simulink model "tarot_replanning2"  (R2022a)
settings: Solver=ode45  StartTime=0.0  StopTime=sim_params.max_sim_time  FixedStep=uav.dynamics_srate  MaxStep=uav.dynamics_srate  MinStep=.005  RelTol=.005
undefined symbols (not defined in the file): constant_x_wind, constant_y_wind, constant_z_wind, DiscIntNeverNeededParam, P_failure, processes, sim_params, trajectory, uav
libraries: shared6dof x1, dspstat3 x1
(part 2 of 2)

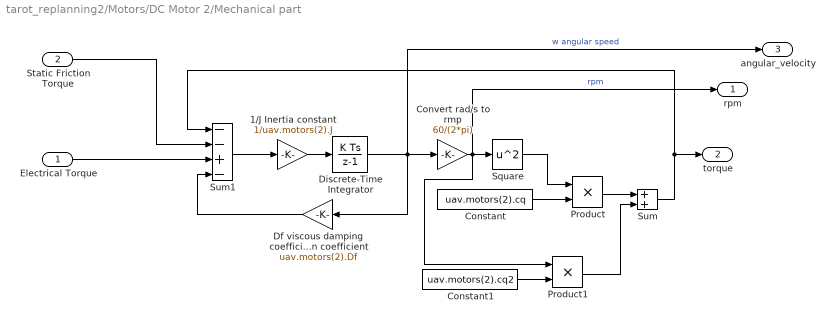
== system tarot_replanning2/Motors/DC Motor 2/Mechanical part ==
  Electrical Torque : Inport
  Static Friction Torque : Inport  Port=2
  1/J Inertia constant : Gain  Gain=1/uav.motors(2).J
  Constant : Constant  Value=uav.motors(2).cq
  Constant1 : Constant  Value=uav.motors(2).cq2
  Convert rad/s to rmp : Gain  Gain=60/(2*pi)
  "Df viscous damping coefficient Dynamic Friction coefficient " : Gain  Gain=uav.motors(2).Df
  Discrete-Time Integrator : DiscreteIntegrator  gainval=1  InitialCondition=sim_params.initial_conditions.w2  SampleTime=uav.dynamics_srate  ICPrevOutput=DiscIntNeverNeededParam  ICPrevScaledInput=DiscIntNeverNeededParam
  Product : Product
  Product1 : Product
  Square : Math  Operator=square
  Sum : Sum
  Sum1 : Sum  Inputs=--+-
  rpm : Outport  VectorParamsAs1DForOutWhenUnconnected=off
  torque : Outport  Port=2
  angular_velocity : Outport  Port=3
  wires:
  1/J Inertia constant/1 -> Discrete-Time Integrator/1
  Static Friction Torque/1 -> Sum1/2
  "Df viscous damping coefficient Dynamic Friction coefficient "/1 -> Sum1/4
  Discrete-Time Integrator/1 -> angular_velocity/1, Convert rad/s to rmp/1, "Df viscous damping coefficient Dynamic Friction coefficient "/1  "w angular speed"
  Sum1/1 -> 1/J Inertia constant/1
  Electrical Torque/1 -> Sum1/3
  Sum/1 -> Sum1/1, torque/1
  Square/1 -> Product/1
  Constant/1 -> Product/2
  Product/1 -> Sum/1
  Constant1/1 -> Product1/2
  Convert rad/s to rmp/1 -> rpm/1, Product1/1, Square/1  "rpm"
  Product1/1 -> Sum/2

== system tarot_replanning2/Motors/DC Motor 3/Electrical part ==
  ESC voltage : Inport
  w angular speed : Inport  Port=2
  1/R : Gain  Gain=1/uav.motors(3).Req
  Ke (Torque constant)1 : Gain  Gain=uav.motors(3).Ke_eq
  Kt (Torque constant) Kt=Ke for an ideal square wave motor : Gain  Gain=uav.motors(3).Ke_eq
  Saturation : Saturate  UpperLimit=uav.motors(3).current_limit  LowerLimit=0
  Sum : Sum  Inputs=|+-
  Electrical Torque : Outport  VectorParamsAs1DForOutWhenUnconnected=off
  current : Outport  Port=2  VectorParamsAs1DForOutWhenUnconnected=off
  wires:
  1/R/1 -> Saturation/1  "current i"
  Sum/1 -> 1/R/1
  Kt (Torque constant) Kt=Ke for an ideal square wave motor/1 -> Electrical Torque/1
  Ke (Torque constant)1/1 -> Sum/2
  ESC voltage/1 -> Sum/1
  w angular speed/1 -> Ke (Torque constant)1/1
  Saturation/1 -> Kt (Torque constant) Kt=Ke for an ideal square wave motor/1, current/1

== system tarot_replanning2/Motors/DC Motor 3/Mechanical part ==
  Electrical Torque : Inport
  Static Friction Torque : Inport  Port=2
  1/J Inertia constant : Gain  Gain=1/uav.motors(3).J
  Constant : Constant  Value=uav.motors(3).cq
  Constant1 : Constant  Value=uav.motors(3).cq2
  Convert rad/s to rmp : Gain  Gain=60/(2*pi)
  "Df viscous damping coefficient Dynamic Friction coefficient " : Gain  Gain=uav.motors(3).Df
  Discrete-Time Integrator : DiscreteIntegrator  gainval=1  InitialCondition=sim_params.initial_conditions.w3  SampleTime=uav.dynamics_srate  ICPrevOutput=DiscIntNeverNeededParam  ICPrevScaledInput=DiscIntNeverNeededParam
  Product : Product
  Product1 : Product
  Square : Math  Operator=square
  Sum : Sum
  Sum1 : Sum  Inputs=--+-
  rpm : Outport  VectorParamsAs1DForOutWhenUnconnected=off
  torque : Outport  Port=2
  angular_velocity : Outport  Port=3
  wires:
  1/J Inertia constant/1 -> Discrete-Time Integrator/1
  Static Friction Torque/1 -> Sum1/2
  "Df viscous damping coefficient Dynamic Friction coefficient "/1 -> Sum1/4
  Discrete-Time Integrator/1 -> angular_velocity/1, "Df viscous damping coefficient Dynamic Friction coefficient "/1, Convert rad/s to rmp/1  "w angular speed"
  Sum1/1 -> 1/J Inertia constant/1
  Electrical Torque/1 -> Sum1/3
  Sum/1 -> torque/1, Sum1/1
  Square/1 -> Product/1
  Constant/1 -> Product/2
  Product/1 -> Sum/1
  Constant1/1 -> Product1/2
  Convert rad/s to rmp/1 -> Product1/1, rpm/1, Square/1  "rpm"
  Product1/1 -> Sum/2

== system tarot_replanning2/Motors/DC Motor 4/Electrical part ==
  ESC voltage : Inport
  w angular speed : Inport  Port=2
  1/R : Gain  Gain=1/uav.motors(4).Req
  Ke (Torque constant)1 : Gain  Gain=uav.motors(4).Ke_eq
  Kt (Torque constant) Kt=Ke for an ideal square wave motor : Gain  Gain=uav.motors(4).Ke_eq
  Saturation : Saturate  UpperLimit=uav.motors(4).current_limit  LowerLimit=0
  Sum : Sum  Inputs=|+-
  Electrical Torque : Outport  VectorParamsAs1DForOutWhenUnconnected=off
  current : Outport  Port=2  VectorParamsAs1DForOutWhenUnconnected=off
  wires:
  1/R/1 -> Saturation/1  "current i"
  Sum/1 -> 1/R/1
  Kt (Torque constant) Kt=Ke for an ideal square wave motor/1 -> Electrical Torque/1
  Ke (Torque constant)1/1 -> Sum/2
  ESC voltage/1 -> Sum/1
  w angular speed/1 -> Ke (Torque constant)1/1
  Saturation/1 -> Kt (Torque constant) Kt=Ke for an ideal square wave motor/1, current/1

== system tarot_replanning2/Motors/DC Motor 4/Mechanical part ==
  Electrical Torque : Inport
  Static Friction Torque : Inport  Port=2
  1/J Inertia constant : Gain  Gain=1/uav.motors(4).J
  Constant : Constant  Value=uav.motors(4).cq
  Constant1 : Constant  Value=uav.motors(4).cq2
  Convert rad/s to rmp : Gain  Gain=60/(2*pi)
  "Df viscous damping coefficient Dynamic Friction coefficient " : Gain  Gain=uav.motors(4).Df
  Discrete-Time Integrator : DiscreteIntegrator  gainval=1  InitialCondition=sim_params.initial_conditions.w4  SampleTime=uav.dynamics_srate  ICPrevOutput=DiscIntNeverNeededParam  ICPrevScaledInput=DiscIntNeverNeededParam
  Product : Product
  Product1 : Product
  Square : Math  Operator=square
  Sum : Sum
  Sum1 : Sum  Inputs=--+-
  rpm : Outport  VectorParamsAs1DForOutWhenUnconnected=off
  torque : Outport  Port=2
  angular_velocity : Outport  Port=3
  wires:
  1/J Inertia constant/1 -> Discrete-Time Integrator/1
  Static Friction Torque/1 -> Sum1/2
  "Df viscous damping coefficient Dynamic Friction coefficient "/1 -> Sum1/4
  Discrete-Time Integrator/1 -> angular_velocity/1, Convert rad/s to rmp/1, "Df viscous damping coefficient Dynamic Friction coefficient "/1  "w angular speed"
  Sum1/1 -> 1/J Inertia constant/1
  Electrical Torque/1 -> Sum1/3
  Sum/1 -> torque/1, Sum1/1
  Square/1 -> Product/1
  Constant/1 -> Product/2
  Product/1 -> Sum/1
  Constant1/1 -> Product1/2
  Convert rad/s to rmp/1 -> rpm/1, Product1/1, Square/1  "rpm"
  Product1/1 -> Sum/2

== system tarot_replanning2/Motors/DC Motor 5/Electrical part ==
  ESC voltage : Inport
  w angular speed : Inport  Port=2
  1/R : Gain  Gain=1/uav.motors(5).Req
  Ke (Torque constant)1 : Gain  Gain=uav.motors(5).Ke_eq
  Kt (Torque constant) Kt=Ke for an ideal square wave motor : Gain  Gain=uav.motors(5).Ke_eq
  Saturation : Saturate  UpperLimit=uav.motors(5).current_limit  LowerLimit=0
  Sum : Sum  Inputs=|+-
  Electrical Torque : Outport  VectorParamsAs1DForOutWhenUnconnected=off
  current : Outport  Port=2  VectorParamsAs1DForOutWhenUnconnected=off
  wires:
  1/R/1 -> Saturation/1  "current i"
  Sum/1 -> 1/R/1
  Kt (Torque constant) Kt=Ke for an ideal square wave motor/1 -> Electrical Torque/1
  Ke (Torque constant)1/1 -> Sum/2
  ESC voltage/1 -> Sum/1
  w angular speed/1 -> Ke (Torque constant)1/1
  Saturation/1 -> Kt (Torque constant) Kt=Ke for an ideal square wave motor/1, current/1

== system tarot_replanning2/Motors/DC Motor 5/Mechanical part ==
  Electrical Torque : Inport
  Static Friction Torque : Inport  Port=2
  1/J Inertia constant : Gain  Gain=1/uav.motors(5).J
  Constant : Constant  Value=uav.motors(5).cq
  Constant1 : Constant  Value=uav.motors(5).cq2
  Convert rad/s to rmp : Gain  Gain=60/(2*pi)
  "Df viscous damping coefficient Dynamic Friction coefficient " : Gain  Gain=uav.motors(5).Df
  Discrete-Time Integrator : DiscreteIntegrator  gainval=1  InitialCondition=sim_params.initial_conditions.w5  SampleTime=uav.dynamics_srate  ICPrevOutput=DiscIntNeverNeededParam  ICPrevScaledInput=DiscIntNeverNeededParam
  Product : Product
  Product1 : Product
  Square : Math  Operator=square
  Sum : Sum
  Sum1 : Sum  Inputs=--+-
  rpm : Outport  VectorParamsAs1DForOutWhenUnconnected=off
  torque : Outport  Port=2
  angular_velocity : Outport  Port=3
  wires:
  1/J Inertia constant/1 -> Discrete-Time Integrator/1
  Static Friction Torque/1 -> Sum1/2
  "Df viscous damping coefficient Dynamic Friction coefficient "/1 -> Sum1/4
  Discrete-Time Integrator/1 -> angular_velocity/1, Convert rad/s to rmp/1, "Df viscous damping coefficient Dynamic Friction coefficient "/1  "w angular speed"
  Sum1/1 -> 1/J Inertia constant/1
  Electrical Torque/1 -> Sum1/3
  Sum/1 -> torque/1, Sum1/1
  Square/1 -> Product/1
  Constant/1 -> Product/2
  Product/1 -> Sum/1
  Constant1/1 -> Product1/2
  Convert rad/s to rmp/1 -> rpm/1, Product1/1, Square/1  "rpm"
  Product1/1 -> Sum/2

== system tarot_replanning2/Motors/DC Motor 6/Electrical part ==
  ESC voltage : Inport
  w angular speed : Inport  Port=2
  1/R : Gain  Gain=1/uav.motors(6).Req
  Ke (Torque constant)1 : Gain  Gain=uav.motors(6).Ke_eq
  Kt (Torque constant) Kt=Ke for an ideal square wave motor : Gain  Gain=uav.motors(6).Ke_eq
  Saturation : Saturate  UpperLimit=uav.motors(6).current_limit  LowerLimit=0
  Sum : Sum  Inputs=|+-
  Electrical Torque : Outport  VectorParamsAs1DForOutWhenUnconnected=off
  current : Outport  Port=2  VectorParamsAs1DForOutWhenUnconnected=off
  wires:
  1/R/1 -> Saturation/1  "current i"
  Sum/1 -> 1/R/1
  Kt (Torque constant) Kt=Ke for an ideal square wave motor/1 -> Electrical Torque/1
  Ke (Torque constant)1/1 -> Sum/2
  ESC voltage/1 -> Sum/1
  w angular speed/1 -> Ke (Torque constant)1/1
  Saturation/1 -> Kt (Torque constant) Kt=Ke for an ideal square wave motor/1, current/1

== system tarot_replanning2/Motors/DC Motor 6/Mechanical part ==
  Electrical Torque : Inport
  Static Friction Torque : Inport  Port=2
  1/J Inertia constant : Gain  Gain=1/uav.motors(6).J
  Constant : Constant  Value=uav.motors(6).cq
  Constant1 : Constant  Value=uav.motors(6).cq2
  Convert rad/s to rmp : Gain  Gain=60/(2*pi)
  "Df viscous damping coefficient Dynamic Friction coefficient " : Gain  Gain=uav.motors(6).Df
  Discrete-Time Integrator : DiscreteIntegrator  gainval=1  InitialCondition=sim_params.initial_conditions.w6  SampleTime=uav.dynamics_srate  ICPrevOutput=DiscIntNeverNeededParam  ICPrevScaledInput=DiscIntNeverNeededParam
  Product : Product
  Product1 : Product
  Square : Math  Operator=square
  Sum : Sum
  Sum1 : Sum  Inputs=--+-
  rpm : Outport  VectorParamsAs1DForOutWhenUnconnected=off
  torque : Outport  Port=2
  angular_velocity : Outport  Port=3
  wires:
  1/J Inertia constant/1 -> Discrete-Time Integrator/1
  Static Friction Torque/1 -> Sum1/2
  "Df viscous damping coefficient Dynamic Friction coefficient "/1 -> Sum1/4
  Discrete-Time Integrator/1 -> angular_velocity/1, "Df viscous damping coefficient Dynamic Friction coefficient "/1, Convert rad/s to rmp/1  "w angular speed"
  Sum1/1 -> 1/J Inertia constant/1
  Electrical Torque/1 -> Sum1/3
  Sum/1 -> torque/1, Sum1/1
  Square/1 -> Product/1
  Constant/1 -> Product/2
  Product/1 -> Sum/1
  Constant1/1 -> Product1/2
  Convert rad/s to rmp/1 -> rpm/1, Product1/1, Square/1  "rpm"
  Product1/1 -> Sum/2

== system tarot_replanning2/Motors/DC Motor 7/Electrical part ==
  ESC voltage : Inport
  w angular speed : Inport  Port=2
  1/R : Gain  Gain=1/uav.motors(7).Req
  Ke (Torque constant)1 : Gain  Gain=uav.motors(7).Ke_eq
  Kt (Torque constant) Kt=Ke for an ideal square wave motor : Gain  Gain=uav.motors(7).Ke_eq
  Saturation : Saturate  UpperLimit=uav.motors(7).current_limit  LowerLimit=0
  Sum : Sum  Inputs=|+-
  Electrical Torque : Outport  VectorParamsAs1DForOutWhenUnconnected=off
  current : Outport  Port=2  VectorParamsAs1DForOutWhenUnconnected=off
  wires:
  1/R/1 -> Saturation/1  "current i"
  Sum/1 -> 1/R/1
  Kt (Torque constant) Kt=Ke for an ideal square wave motor/1 -> Electrical Torque/1
  Ke (Torque constant)1/1 -> Sum/2
  ESC voltage/1 -> Sum/1
  w angular speed/1 -> Ke (Torque constant)1/1
  Saturation/1 -> Kt (Torque constant) Kt=Ke for an ideal square wave motor/1, current/1

== system tarot_replanning2/Motors/DC Motor 7/Mechanical part ==
  Electrical Torque : Inport
  Static Friction Torque : Inport  Port=2
  1/J Inertia constant : Gain  Gain=1/uav.motors(7).J
  Constant : Constant  Value=uav.motors(7).cq
  Constant1 : Constant  Value=uav.motors(7).cq2
  Convert rad/s to rmp : Gain  Gain=60/(2*pi)
  "Df viscous damping coefficient Dynamic Friction coefficient " : Gain  Gain=uav.motors(7).Df
  Discrete-Time Integrator : DiscreteIntegrator  gainval=1  InitialCondition=sim_params.initial_conditions.w7  SampleTime=uav.dynamics_srate  ICPrevOutput=DiscIntNeverNeededParam  ICPrevScaledInput=DiscIntNeverNeededParam
  Product : Product
  Product1 : Product
  Square : Math  Operator=square
  Sum : Sum
  Sum1 : Sum  Inputs=--+-
  rpm : Outport  VectorParamsAs1DForOutWhenUnconnected=off
  torque : Outport  Port=2
  angular_velocity : Outport  Port=3
  wires:
  1/J Inertia constant/1 -> Discrete-Time Integrator/1
  Static Friction Torque/1 -> Sum1/2
  "Df viscous damping coefficient Dynamic Friction coefficient "/1 -> Sum1/4
  Discrete-Time Integrator/1 -> "Df viscous damping coefficient Dynamic Friction coefficient "/1, angular_velocity/1, Convert rad/s to rmp/1  "w angular speed"
  Sum1/1 -> 1/J Inertia constant/1
  Electrical Torque/1 -> Sum1/3
  Sum/1 -> torque/1, Sum1/1
  Square/1 -> Product/1
  Constant/1 -> Product/2
  Product/1 -> Sum/1
  Constant1/1 -> Product1/2
  Convert rad/s to rmp/1 -> rpm/1, Product1/1, Square/1  "rpm"
  Product1/1 -> Sum/2

== system tarot_replanning2/Motors/DC Motor 8/Electrical part ==
  ESC voltage : Inport
  w angular speed : Inport  Port=2
  1/R : Gain  Gain=1/uav.motors(8).Req
  Ke (Torque constant)1 : Gain  Gain=uav.motors(8).Ke_eq
  Kt (Torque constant) Kt=Ke for an ideal square wave motor : Gain  Gain=uav.motors(8).Ke_eq
  Saturation : Saturate  UpperLimit=uav.motors(8).current_limit  LowerLimit=0
  Sum : Sum  Inputs=|+-
  Electrical Torque : Outport  VectorParamsAs1DForOutWhenUnconnected=off
  current : Outport  Port=2  VectorParamsAs1DForOutWhenUnconnected=off
  wires:
  1/R/1 -> Saturation/1  "current i"
  Sum/1 -> 1/R/1
  Kt (Torque constant) Kt=Ke for an ideal square wave motor/1 -> Electrical Torque/1
  Ke (Torque constant)1/1 -> Sum/2
  ESC voltage/1 -> Sum/1
  w angular speed/1 -> Ke (Torque constant)1/1
  Saturation/1 -> Kt (Torque constant) Kt=Ke for an ideal square wave motor/1, current/1

== system tarot_replanning2/Motors/DC Motor 8/Mechanical part ==
  Electrical Torque : Inport
  Static Friction Torque : Inport  Port=2
  1/J Inertia constant : Gain  Gain=1/uav.motors(3).J
  Constant : Constant  Value=uav.motors(3).cq
  Constant1 : Constant  Value=uav.motors(3).cq2
  Convert rad/s to rmp : Gain  Gain=60/(2*pi)
  "Df viscous damping coefficient Dynamic Friction coefficient " : Gain  Gain=uav.motors(3).Df
  Discrete-Time Integrator : DiscreteIntegrator  gainval=1  InitialCondition=sim_params.initial_conditions.w3  SampleTime=uav.dynamics_srate  ICPrevOutput=DiscIntNeverNeededParam  ICPrevScaledInput=DiscIntNeverNeededParam
  Product : Product
  Product1 : Product
  Square : Math  Operator=square
  Sum : Sum
  Sum1 : Sum  Inputs=--+-
  rpm : Outport  VectorParamsAs1DForOutWhenUnconnected=off
  torque : Outport  Port=2
  angular_velocity : Outport  Port=3
  wires:
  1/J Inertia constant/1 -> Discrete-Time Integrator/1
  Static Friction Torque/1 -> Sum1/2
  "Df viscous damping coefficient Dynamic Friction coefficient "/1 -> Sum1/4
  Discrete-Time Integrator/1 -> angular_velocity/1, Convert rad/s to rmp/1, "Df viscous damping coefficient Dynamic Friction coefficient "/1  "w angular speed"
  Sum1/1 -> 1/J Inertia constant/1
  Electrical Torque/1 -> Sum1/3
  Sum/1 -> torque/1, Sum1/1
  Square/1 -> Product/1
  Constant/1 -> Product/2
  Product/1 -> Sum/1
  Constant1/1 -> Product1/2
  Convert rad/s to rmp/1 -> rpm/1, Product1/1, Square/1  "rpm"
  Product1/1 -> Sum/2

== matlab function tarot_replanning2/ESCs/ESC1/reduced output fault ==
  data: Pf input; p input; u input; y output; s output
function [y, s]= reduced_output_fault(Pf, p, u)

if p <= Pf
    y = u * interp1([0.0 1.0],[1.05 .895],Pf*.8);
    y = min(u*.995, y);
    s = 1;
else
    y = u;
    s = 0;
end

== matlab function tarot_replanning2/ESCs/ESC3/reduced output fault ==
  data: Pf input; p input; u input; y output; s output
function [y, s]= reduced_output_fault(Pf, p, u)

if p <= Pf
    y = u * interp1([0.0 1.0],[1.005 .885],Pf);
    s = 1;
else
    y = u;
    s = 0;
end

== matlab function tarot_replanning2/Battery/MATLAB Function1 ==
  settings: updateMethod=DISCRETE  sampleTime=.2
  data: mu input; y output; sigma input
function y = addNoise(mu, sigma)

y = normrnd(mu, sigma);

== matlab function tarot_replanning2/ESCs/ESC4/reduced output fault ==
  data: Pf input; p input; u input; y output; s output
function [y, s]= reduced_output_fault(Pf, p, u)

if p <= Pf
    y = u * interp1([0.0 1.0],[1.005 .885],Pf);
    s = 1;
else
    y = u;
    s = 0;
end

== matlab function tarot_replanning2/ESCs/ESC5/reduced output fault ==
  data: Pf input; p input; u input; y output; s output
function [y, s]= reduced_output_fault(Pf, p, u)

if p <= Pf
    y = u * interp1([0.0 1.0],[1.005 .885],Pf);
    s = 1;
else
    y = u;
    s = 0;
end

== matlab function tarot_replanning2/ESCs/ESC6/reduced output fault ==
  data: Pf input; p input; u input; y output; s output
function [y, s]= reduced_output_fault(Pf, p, u)

if p <= Pf
    y = u * interp1([0.0 1.0],[1.005 .885],Pf);
    s = 1;
else
    y = u;
    s = 0;
end

== matlab function tarot_replanning2/ESCs/ESC7/reduced output fault ==
  data: Pf input; p input; u input; y output; s output
function [y, s]= reduced_output_fault(Pf, p, u)

if p <= Pf
    y = u * interp1([0.0 1.0],[1.005 .885],Pf);
    s = 1;
else
    y = u;
    s = 0;
end

== matlab function tarot_replanning2/ESCs/ESC8/reduced output fault ==
  data: Pf input; p input; u input; y output; s output
function [y, s]= reduced_output_fault(Pf, p, u)

if p <= Pf
    y = u * interp1([0.0 1.0],[1.005 .885],Pf);
    s = 1;
else
    y = u;
    s = 0;
end

== matlab function tarot_replanning2/Control allocation1 ==
  data: Fx input; wref1 output; Fy input; Fz input; Troll input; Tpitch input; Tyaw input; wref2 output; wref3 output; wref4 output; wref5 output; wref6 output; wref7 output; wref8 output; Vbat input
function [wref1,wref2,wref3,wref4,wref5,wref6,wref7,wref8] = fcn(Fx,Fy,Fz,Troll,Tpitch,Tyaw,Vbat)
%% parameters 
%Maximum speed that the motors can reach in rad/s
Max_speed=670; %668.11
%Max total Thrust all motors can generate in N
Max_thrust=352; %351.451
%Max torque in each individual axis



% arm length - distances from the octorotor center of mass ...
%        to the center of mass of all its rotors are equal and denoted by l.
l=0.635;
% thrust motor constant [Ns^2/rad^2]
b=9.8419e-05; % 
% rotor drag constant [Nms^2/rad^2]
d=1.8503e-06; % 

%angles
angsm=cos(pi/8); % 22.5 
anglg=cos(3*pi/8); % 67.5

% control allocation matrix
A_f=[b b b b b b b b; ...
    b*l*anglg b*l*angsm -b*l*angsm -b*l*anglg -b*l*anglg -b*l*angsm b*l*angsm b*l*anglg; ...
    -b*l*angsm -b*l*anglg -b*l*anglg -b*l*angsm b*l*angsm b*l*anglg b*l*anglg b*l*angsm; ...
    d -d d -d d -d d -d];

% duty cycle initialization
DC=zeros(8,1);

%desired input
u_des=[Fz;Troll;Tpitch;Tyaw];

%control allocation
Omega_s=pinv(A_f)*u_des; %inverse of A_f is A_f\

% velocity checking
wref=zeros(8,1);
for i=1:length(Omega_s)
    if Omega_s(i)<0
        wref(i)=0;
    elseif Omega_s(i)>Max_speed^2
        wref(i)=Max_speed;
    else
        wref(i)=sqrt(Omega_s(i));
    end
end

%velocity assignment in V
DCfactor=0.001355; %original direct conversion multiply=0.0325; wref(i)=wref(i)*multiply;
Voltconversion=0.0325;

% "virtual" ESC 
for i=1:length(wref)
    % voltage saturation check
    if(wref(i)*DCfactor*Vbat > Vbat)
        wref(i)=Vbat;
        DC(i)=1;
    elseif(wref(i)*DCfactor*Vbat <=0)
        wref(i)=0.065;
        DC(i)=0.01;
    else
        DC(i)=wref(i)*DCfactor;
        %wref(i)=Vbat*DC(i); 
        wref(i)=wref(i)*Voltconversion;
    end
end

wref1=wref(1);
wref2=wref(2);
wref3=wref(3);
wref4=wref(4);
wref5=wref(5);
wref6=wref(6);
wref7=wref(7);
wref8=wref(8);


end

== matlab function tarot_replanning2/GPS1/measurement ==
  data: u input; y output; t input
function y = gps_measurement(u,t)
if t< 5.0
    see=1;
end
y = zeros(6,1);
posnoisestd=0.2; 
velnoisestd=0.02;
%imunoisestd=.00001;
noisepos=posnoisestd.*randn(3,1);
noisevel=velnoisestd.*randn(3,1);
%noiseimu=imunoisestd.*randn(3,1);
noise=[noisepos ;noisevel];%; noiseimu];
y = y + u + noise;

== matlab function tarot_replanning2/Battery/MATLAB Function ==
  data: u input; x output; u1 input; pos input; u output; trajectory parameter; triggered input; triggered output
function [x, u, triggered] = fcn(u, u1, pos, trajectory, triggered)
    
    if  abs(u - u1) > 1.5 && triggered == 0
        x = 1;
        trajectory.start = pos(1:2)';
        triggered = 1;
    else
        x = 0;
    end

== matlab function tarot_replanning2/Forces and Moments Calculation ==
  data: w1 input; Fx output; w2 input; w3 input; w4 input; w5 input; w6 input; Fy output; Fz output; Mx output; My output; Mz output; w7 input; w8 input; Phi input; The input; Psi input; disturbance input
function [Fx,Fy,Fz,Mx,My,Mz] = fcn(w1,w2,w3,w4,w5,w6,w7,w8,Phi,The,Psi, disturbance)
octomodel.g=9.80;
octomodel.m_t=10.66;
octomodel.l=0.635;
% Phi,The,Psi, in rad
w  = [w1; w2; w3; w4;w5; w6; w7; w8];

%% not used
%to fix numerical issues
%w=round(w,2);
% transform rpm to rad/s
%w=w./(60/(2*pi));

%% thrust generated by rotors

% Approach 1
% coef_t = 0.065;
%thrust = coef_t * density of air * velocity^2 * propeller diameter (m) ^4
%velocity in rev/sec, where  1 rev/sec = 1 rpm/60
%T = coef_t*1.225*((w./60).^2)*.47^4; % 18.5 inches ~ 0.47 m

% Approach 2
% thrust motor constant [Ns^2/rad^2]
b=9.8419e-05; % 
T = b.*((2*pi).*w./60).^2;

% total thrust generated by rotors
T_total=sum(T);
T_total=round(T_total*100)/100;

%% Forces in the local frame 
R_b_e = [cos(Psi)*cos(The) cos(Psi)*sin(The)*sin(Phi)-sin(Psi)*cos(Phi) cos(Psi)*sin(The)*cos(Phi)+sin(Psi)*sin(Phi);
       sin(Psi)*cos(The) sin(Psi)*sin(The)*sin(Phi)+cos(Psi)*cos(Phi) sin(Psi)*sin(The)*cos(Phi)-cos(Psi)*sin(Phi);
       -sin(The)         cos(The)*sin(Phi)                            cos(The)*cos(Phi)]; % Rib

Ftot_b=R_b_e'*[0 ;0; -octomodel.m_t*octomodel.g]+[0; 0; T_total]+disturbance; 
Fx=Ftot_b(1);Fy=Ftot_b(2);Fz=Ftot_b(3);

%% Moments in the local frame 
% moment of each rotor
% Approach 1
%M = (2.138e-08)*w.^2 + (-1.279e-05)*w ;

% Approach 2
% rotor drag constant [Nms^2/rad^2]
d=1.8503e-06; % 
M = d.*((2*pi).*w./60).^2;


% torque generated by rotors
%motor angles
angsm=cos(pi/8); % 22.5 
anglg=cos(3*pi/8); % 67.5

Mx=octomodel.l*(T(1)*anglg +T(2)*angsm -T(3)*angsm -T(4)*anglg -T(5)*anglg ...
    -T(6)*angsm +T(7)*angsm +T(8)*anglg);%Tau_roll

My=octomodel.l*(-T(1)*angsm -T(2)*anglg -T(3)*anglg -T(4)*angsm +T(5)*angsm ...
    +T(6)*anglg +T(7)*anglg +T(8)*angsm);%Tau_theta

Mz= M(1) -M(2) +M(3) -M(4) +M(5) -M(6) +M(7) -M(8);%%Tau_yaw
end

== matlab function tarot_replanning2/ESCs/ESC2/reduced output fault ==
  data: Pf input; p input; u input; y output; s output
function [y, s]= reduced_output_fault(Pf, p, u)

if p <= Pf
    y = u * interp1([0.0 1.0],[1.005 .885],Pf);
    s = 1;
else
    y = u;
    s = 0;
end

== stateflow chart tarot_replanning2/Monitors/takeoff and landing ==
  state takeoff
    % take 10 seconds to reach altitude
    du:
    Z_ref = z_setpoint * t / 10;
    t = clock;
  state normal
    du:
    if (abs(pos_vel(1) - trajectory.waypoints(waypoint,1)) < 3.5 && abs(pos_vel(2) - trajectory.waypoints(waypoint,2)) < 3.5)
    waypoint = waypoint + 1;
    end
  state land
    du:
    if (abs(pos_vel(1) - trajectory.destination(1,1)) < 10 && abs(pos_vel(2) - trajectory.destination(1,2) < 10))
    Z_ref = 0;
    end
    if (pos_vel(3) < 1 && Z_ref < 1)
    stop = true;
    end
    if (abs(pos_vel(1) - trajectory.destination(1,1)) < 2 && abs(pos_vel(2) - trajectory.destination(1,2) < 2))
    stop = true;
    end
  (default) -> takeoff : {stop = false; t = clock; }
  takeoff -> normal : [pos_vel(3) >= .9*z_setpoint ]
      | {Z_ref = z_setpoint; waypoint = 2; }
  normal -> land : [waypoint == length(trajectory.waypoints)+1]{waypoint = 0;}
  data: waypoint output; pos_vel input; Z_ref output; trajectory parameter; stop output boolean; z_setpoint input; clock input; t local

== stateflow chart tarot_replanning2/Monitors/position error calc ==
  state calc_pos_err
    adj = .95;
    dv = abs(sqrt(pos_vel(4)^2 + pos_vel(5)^2) -  1);
    pos_err = abs(sqrt((abs(pos_vel(1) - x_ref)*adj)^2 + abs((pos_vel(2) - y_ref)*adj)^2) - .5*dv);
    x_pos_err = pos_vel(1) - x_ref;
    y_pos_err = pos_vel(2) - y_ref;
  (default) -> calc_pos_err
  data: pos_vel input; x_ref input; y_ref input; pos_err output; dv local; adj local; x_pos_err output; y_pos_err output
